simulink model "robotdynamic_path_simulink"  (R2018b)
settings: Solver=VariableStepAuto  StartTime=0.0  StopTime=10.0  RelTol=1e-3
values from neighbouring files (symbols this model uses):
  alpha = (1-learning_rate)*alpha + (learning_rate)*alpha_episode    [controlWithLearnedSlipModel.m]
  axel_len = .62    (= 0.62)    [controlWithLearnedSlipModel.m]    (also in run_model.m; wheelaccelDynamics.m)
  curve = (1 - t).^3 .* P0          + 3*(1-t).^2 .*t .* P1          + 3*(1-t).*t.^2 .* P2          + t.^3 .* P3    [controlWithLearnedSlipModel.m]
  omega_dx = delta_theta_delta_t ./ delta_x_delta_t    [controlWithLearnedSlipModel.m]
  path_fwd = 1    [controlWithLearnedSlipModel.m]
settings Model: Creator=fworg  LastModifiedBy=fworg

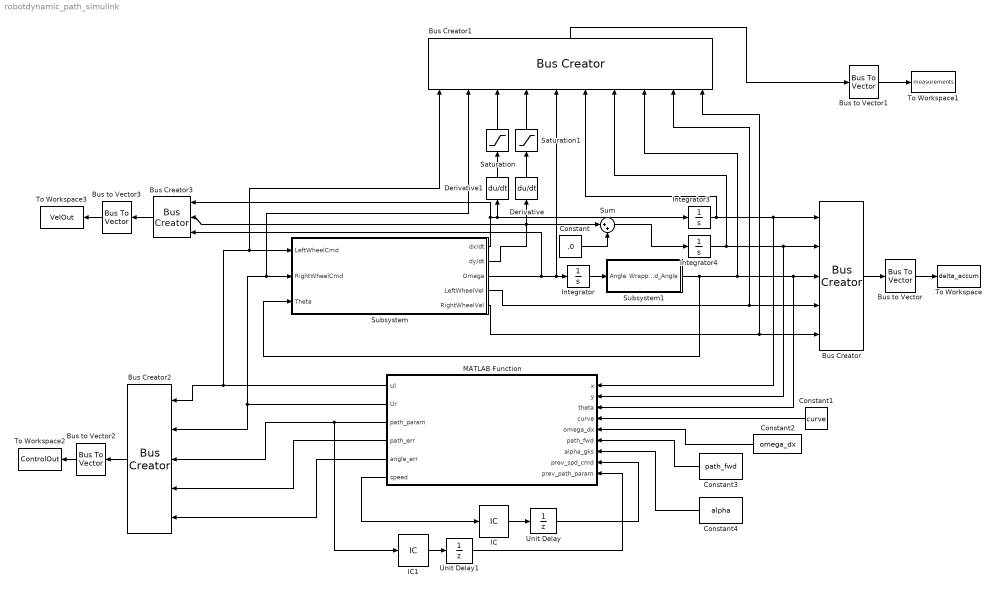
== system robotdynamic_path_simulink ==
  Bus Creator : BusCreator  Inputs=5
  Bus Creator1 : BusCreator  Inputs=10
  Bus Creator2 : BusCreator  Inputs=5
  Bus Creator3 : BusCreator  Inputs=3
  Bus to Vector{,1..3} (4 alike) : BusToVector
  Constant : Constant  Value=.0
  Constant1 : Constant  Value=curve
  Constant2 : Constant  Value=omega_dx
  Constant3 : Constant  Value=path_fwd
  Constant4 : Constant  Value=alpha
  Derivative : Derivative
  Derivative1 : Derivative
  IC : InitialCondition  Value=0
  IC1 : InitialCondition  Value=0
  Integrator : Integrator
  Integrator3 : Integrator
  Integrator4 : Integrator
  MATLAB Function : MATLAB Function  TreatAsAtomicUnit=on
  Saturation : Saturate  UpperLimit=1  LowerLimit=-1
  Saturation1 : Saturate  UpperLimit=1  LowerLimit=-1
  Subsystem : Subsystem
  Subsystem1 : Subsystem
  Sum : Sum  Inputs=|++
  To Workspace : ToWorkspace  VariableName=delta_accum  SaveFormat=Timeseries  SampleTime=-1
  To Workspace1 : ToWorkspace  VariableName=measurements  SaveFormat=Timeseries  SampleTime=-1
  To Workspace2 : ToWorkspace  VariableName=ControlOut  SaveFormat=Timeseries  SampleTime=-1
  To Workspace3 : ToWorkspace  VariableName=VelOut  SaveFormat=Timeseries  SampleTime=-1
  Unit Delay : UnitDelay  SampleTime=-1
  Unit Delay1 : UnitDelay  SampleTime=-1
  wires:
  Subsystem/3(Omega) -> Bus Creator3/3, Bus Creator1/5, Integrator/1
  Subsystem/4(LeftWheelVel) -> Bus Creator/4, Bus Creator1/9
  Subsystem/5(RightWheelVel) -> Bus Creator/5, Bus Creator1/10
  Bus Creator/1 -> Bus to Vector/1
  Bus to Vector/1 -> To Workspace/1
  Integrator/1 -> Subsystem1/1(Angle)
  Subsystem1/1(Wrapped_Angle) -> Subsystem/3(Theta), MATLAB Function/3(theta), Bus Creator/3, Bus Creator1/8
  Integrator4/1 -> MATLAB Function/2(y), Bus Creator/2, Bus Creator1/7
  Bus Creator1/1 -> Bus to Vector1/1
  Subsystem/1(dx/dt) -> Bus Creator3/1, Derivative1/1, Integrator3/1
  Subsystem/2(dy/dt) -> Bus Creator3/2, Sum/1, Derivative/1
  Integrator3/1 -> Bus Creator1/6, MATLAB Function/1(x), Bus Creator/1
  Bus to Vector1/1 -> To Workspace1/1
  Derivative/1 -> Saturation1/1
  Derivative1/1 -> Saturation/1
  Saturation/1 -> Bus Creator1/3
  Saturation1/1 -> Bus Creator1/4
  Constant/1 -> Sum/2
  Sum/1 -> Integrator4/1
  MATLAB Function/6(speed) -> IC/1
  MATLAB Function/3(path_param) -> IC1/1, Bus Creator2/3
  IC/1 -> Unit Delay/1
  IC1/1 -> Unit Delay1/1
  Constant1/1 -> MATLAB Function/4(curve)
  Constant3/1 -> MATLAB Function/6(path_fwd)
  Constant2/1 -> MATLAB Function/5(omega_dx)
  Bus Creator2/1 -> Bus to Vector2/1
  Bus to Vector2/1 -> To Workspace2/1
  MATLAB Function/4(path_err) -> Bus Creator2/4
  MATLAB Function/5(angle_err) -> Bus Creator2/5
  Bus to Vector3/1 -> To Workspace3/1
  Bus Creator3/1 -> Bus to Vector3/1
  Constant4/1 -> MATLAB Function/7(alpha_gks)
  MATLAB Function/1(Ul) -> Bus Creator1/1, Subsystem/1(LeftWheelCmd), Bus Creator2/1
  MATLAB Function/2(Ur) -> Bus Creator2/2, Bus Creator1/2, Subsystem/2("RightWheelCmd ")
  Unit Delay/1 -> MATLAB Function/8(prev_spd_cmd)
  Unit Delay1/1 -> MATLAB Function/9(prev_path_param)

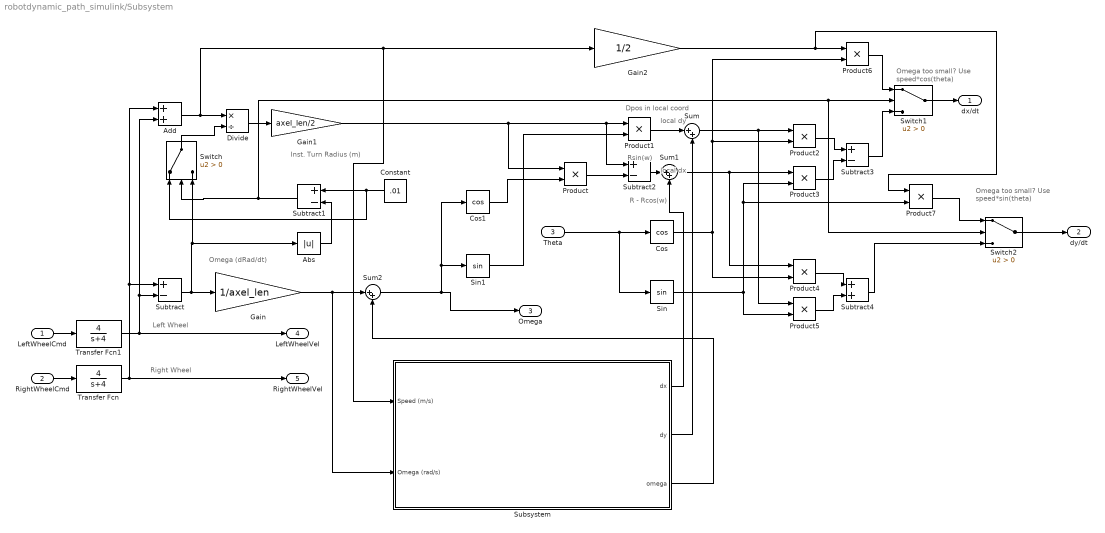
== system robotdynamic_path_simulink/Subsystem ==
  note: Rsin(w)
  note: R - Rcos(w)
  note: Dpos in local coord
  note: Right Wheel
  note: Left Wheel
  note: Omega (dRad/dt)
  note: Inst. Turn Radius (m)
  note: Omega too small?
      | Use speed*cos(theta)
  note: Omega too small?
      | Use speed*sin(theta)
  note: local dx
  note: local dy
  LeftWheelCmd : Inport
  "RightWheelCmd " : Inport  Port=2
  Theta : Inport  Port=3
  Abs : Abs
  Add : Sum
  Constant : Constant  Value=.01
  Cos : Trigonometry  Operator=cos
  Cos1 : Trigonometry  Operator=cos
  Divide : Product  Inputs=*/
  Gain : Gain  Gain=1/axel_len
  Gain1 : Gain  Gain=axel_len/2
  Gain2 : Gain  Gain=1/2
  Product{,1..7} (8 alike) : Product
  Sin : Trigonometry
  Sin1 : Trigonometry
  Subsystem : Subsystem
  Subtract{,1..3} (4 alike) : Sum  Inputs=+-
  Subtract4 : Sum
  Sum : Sum  Inputs=|++
  Sum1 : Sum  Inputs=|++
  Sum2 : Sum  Inputs=|++
  Switch : Switch  Criteria=u2 > Threshold
  Switch1 : Switch  Criteria=u2 > Threshold
  Switch2 : Switch  Criteria=u2 > Threshold
  Transfer Fcn : TransferFcn  Numerator=[4]  Denominator=[1 4]  ContinuousStateAttributes='rightWheel'
  Transfer Fcn1 : TransferFcn  Numerator=[4]  Denominator=[1 4]  ContinuousStateAttributes='leftWheel'
  dx/dt : Outport
  dy/dt : Outport  Port=2
  Omega : Outport  Port=3
  LeftWheelVel : Outport  Port=4
  RightWheelVel : Outport  Port=5
  wires:
  "RightWheelCmd "/1 -> Transfer Fcn/1
  LeftWheelCmd/1 -> Transfer Fcn1/1
  Transfer Fcn1/1 -> LeftWheelVel/1, Add/2, Subtract/2
  Transfer Fcn/1 -> RightWheelVel/1, Add/1, Subtract/1
  Subtract/1 -> Switch/3, Abs/1, Gain/1
  Add/1 -> Subsystem/1(Speed (m/s)), Gain2/1, Divide/1
  Divide/1 -> Gain1/1
  Cos1/1 -> Product/2
  Sin1/1 -> Product1/2
  Switch/1 -> Divide/2
  Constant/1 -> Subtract1/1, Switch/1
  Subtract1/1 -> Switch1/2, Switch2/2, Switch/2
  Abs/1 -> Subtract1/2
  Product/1 -> Subtract2/2
  Theta/1 -> Sin/1, Cos/1
  Sin/1 -> Product5/2, Product7/2, Product3/2
  Product2/1 -> Subtract3/1
  Product3/1 -> Subtract3/2
  Product5/1 -> Subtract4/2
  Product4/1 -> Subtract4/1
  Gain1/1 -> Product/1, Product1/1, Subtract2/1
  Switch2/1 -> dy/dt/1
  Subtract4/1 -> Switch2/3
  Switch1/1 -> dx/dt/1
  Subtract3/1 -> Switch1/3
  Product7/1 -> Switch2/1
  Product6/1 -> Switch1/1
  Cos/1 -> Product6/2, Product2/2, Product4/2
  Gain2/1 -> Product7/1, Product6/1
  Product1/1 -> Sum/1
  Sum/1 -> Product5/1, Product2/1
  Subtract2/1 -> Sum1/1
  Sum1/1 -> Product4/1, Product3/1
  Gain/1 -> Subsystem/2(Omega (rad/s)), Sum2/1
  Sum2/1 -> Cos1/1, Sin1/1, Omega/1
  Subsystem/1(dx) -> Sum1/2
  Subsystem/2("dy ") -> Sum/2
  Subsystem/3("omega ") -> Sum2/2

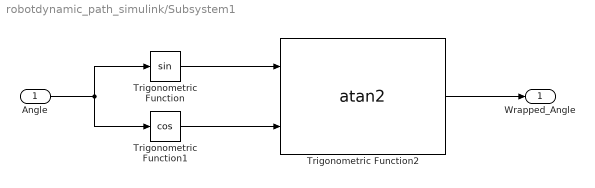
== system robotdynamic_path_simulink/Subsystem1 ==
  Angle : Inport
  Trigonometric Function : Trigonometry
  Trigonometric Function1 : Trigonometry  Operator=cos
  Trigonometric Function2 : Trigonometry  Operator=atan2
  Wrapped_Angle : Outport
  wires:
  Angle/1 -> Trigonometric Function1/1, Trigonometric Function/1
  Trigonometric Function1/1 -> Trigonometric Function2/2
  Trigonometric Function/1 -> Trigonometric Function2/1
  Trigonometric Function2/1 -> Wrapped_Angle/1

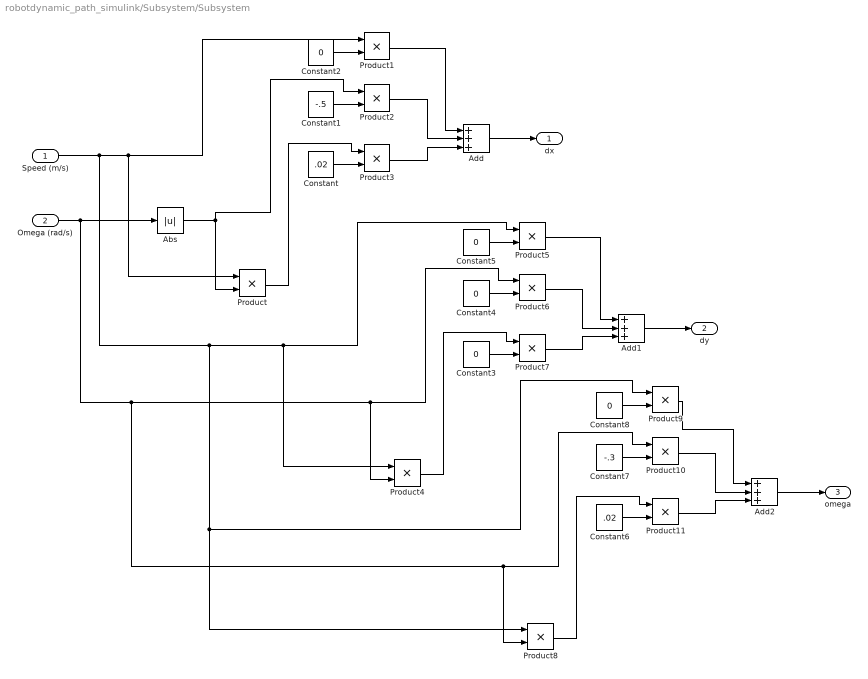
== system robotdynamic_path_simulink/Subsystem/Subsystem ==
  Speed (m/s) : Inport
  Omega (rad/s) : Inport  Port=2
  Abs : Abs
  Add : Sum  Inputs=3
  Add1 : Sum  Inputs=3
  Add2 : Sum  Inputs=3
  Constant : Constant  Value=.02
  Constant1 : Constant  Value=-.5
  Constant{2..5,8} (5 alike) : Constant  Value=0
  Constant6 : Constant  Value=.02
  Constant7 : Constant  Value=-.3
  Product{,1..11} (12 alike) : Product
  dx : Outport
  "dy " : Outport  Port=2
  "omega " : Outport  Port=3
  wires:
  Product/1 -> Product3/1
  Constant/1 -> Product3/2
  Constant1/1 -> Product2/2
  Constant2/1 -> Product1/2
  Abs/1 -> Product2/1, Product/2
  Product3/1 -> Add/3
  Product2/1 -> Add/2
  Product1/1 -> Add/1
  Add/1 -> dx/1
  Add1/1 -> "dy "/1
  Product6/1 -> Add1/2
  Constant3/1 -> Product7/2
  Constant4/1 -> Product6/2
  Product7/1 -> Add1/3
  Product5/1 -> Add1/1
  Constant5/1 -> Product5/2
  Product4/1 -> Product7/1
  Add2/1 -> "omega "/1
  Product8/1 -> Product11/1
  Speed (m/s)/1 -> Product1/1, Product/1, Product8/1, Product9/1, Product5/1, Product4/1
  Product9/1 -> Add2/1
  Product10/1 -> Add2/2
  Constant7/1 -> Product10/2
  Constant8/1 -> Product9/2
  Product11/1 -> Add2/3
  Omega (rad/s)/1 -> Product8/2, Product10/1, Product4/2, Product6/1, Abs/1
  Constant6/1 -> Product11/2

== matlab function robotdynamic_path_simulink/MATLAB Function ==
  data: x input; Ul output size=1; y input; theta input; curve input; omega_dx input; path_fwd input; alpha_gks input; prev_spd_cmd input; Ur output size=1; path_param output size=1; prev_path_param input; path_err output size=1; angle_err output size=1; speed output size=1
function [Ul, Ur, path_param, path_err, angle_err, speed] = PathControl(x, y, theta, curve, omega_dx, path_fwd, alpha_gks, prev_spd_cmd, prev_path_param)
prev_CPP_t = prev_path_param;
axel_len = .62;
top_wheel_speed = 1.0;
[CPP_t, path_err, angle_err] = findCPP2019Spring(x, y, theta, curve, path_fwd);
        if CPP_t < prev_CPP_t
            CPP_t = prev_CPP_t;
        elseif CPP_t > prev_CPP_t
            CPP_t = min(CPP_t, 99);
        end
        path_param = min(99,max(CPP_t,1));
    if path_param <= 96
        steering_lim = 40;
        %omega_dx = 
        speed_setpoint = 1.0;
        angle_gain = 4*2.5;%2.5;
        path_gain  = 3*5.3;%5.3;
        disturbance_gain = 3.0;
        speed_gain = .15;
        steering = min(steering_lim,max(-steering_lim,...
                   omega_dx(int32(path_param)))); %get from path (omega_dx at t)
        speed = prev_spd_cmd;
        speed = speed - speed_gain*(speed - max(.05,min(speed_setpoint)));% todo, limit wheel sped,...
                                            %.5*(left_max_end_speed + right_max_end_speed))));
        p_steering_cmd = -angle_gain*angle_err;
        path_err_comp = path_gain*path_err;
        Ul = 0;
        Ur = 0;
        overall_steering_cmd = steering - 1*p_steering_cmd - 1*path_err_comp;
        omega = speed*overall_steering_cmd;
        speed_gks_comp = (speed - alpha_gks(2) * abs(omega) - alpha_gks(3)*(speed*abs(omega)))...
                         /(1+ alpha_gks(1));
        omega_gks_comp = (omega - alpha_gks(7)*speed)...
                        /(1 +alpha_gks(8) + alpha_gks(9)*speed);
        dist_gks = alpha_gks(4)*speed +alpha_gks(5)*omega + alpha_gks(6)*speed*omega;
        omega_gks_comp = omega_gks_comp - disturbance_gain*dist_gks;
        steering_gks_comp = omega_gks_comp/speed_gks_comp; %is this right?
        [Ul, Ur] = sscv2019Spring(speed_gks_comp, steering_gks_comp,...
                                  axel_len, top_wheel_speed); 
     else
        Ul = 0;
        Ur = 0;
        path_err = 0;
        angle_err= 0;
        speed = 0;
        path_param = 100;
     end
end
